simulink model "ss_series_simulink"  (R2022b)
settings: Solver=VariableStepAuto  StartTime=0.0  StopTime=7  RelTol=1e-3
libraries: MainLibrary x1
settings Model: Creator=cotti  LastModifiedBy=cotti

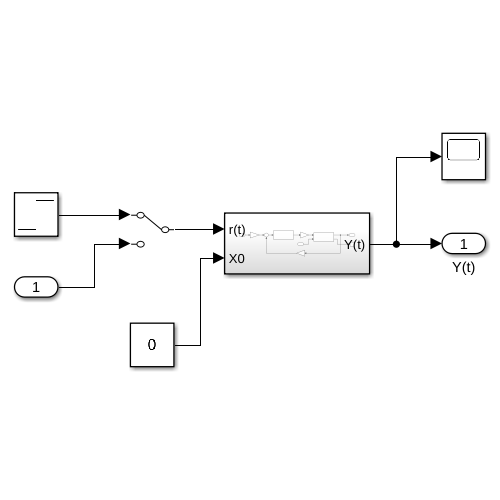
[thumbnail: Simulink's stored preview of the top-level diagram]
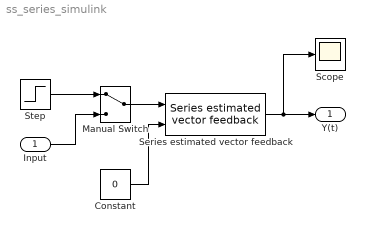
== system ss_series_simulink ==
  Input : Inport
  Constant : Constant  Value=0
  Manual Switch : ManualSwitch
  Scope : Scope
  Series estimated vector feedback : MainLibrary/Series estimated vector feedback  SystemSampleTime=-1  VariantActivationTime=update diagram  Latency=0  AutoFrameSizeCalculation=off
      settings: SourceProductName=Control Cotti
  Step : Step  Time=0  SampleTime=0
  Y(t) : Outport
  wires:
  Manual Switch/1 -> Series estimated vector feedback/1
  Step/1 -> Manual Switch/1
  Input/1 -> Manual Switch/2
  Series estimated vector feedback/1 -> Scope/1, Y(t)/1
  Constant/1 -> Series estimated vector feedback/2
